simulink model "Sample594"  (R2021b)
settings: Solver=VariableStepAuto  StartTime=0.0  StopTime=10.0  RelTol=1e-3
undefined symbols (not defined in the file): DiscIntNeverNeededParam, magnitude, Newton, Raphson
libraries: simulink x402, pid_lib x98
(part 3 of 14)

== system Sample594/cfblk5/cfblk8/cfblk8 ==
  cfblk1 : Inport
  cfblk12 : Inport  Port=2
  cfblk10 : Subsystem
  cfblk11 : If  IfExpression=u1 >= 0  SampleTime=1
  cfblk13 : Subsystem  TreatAsAtomicUnit=on
  cfblk14 : Subsystem  TreatAsAtomicUnit=on
  cfblk{15..21} (7 alike) : Delay  SampleTime=1
  cfblk3 : simulink/Discrete/Difference  ICPrevInput=0.0  OutMin=[]  OutMax=[]  OutDataTypeStr=Inherit: Inherit via back propagation  OutDataType=fixdt(1, 16)  OutScaling=2^-10  DoSatur=off
  cfblk4 : UnitDelay  HasFrameUpgradeWarning=on
  cfblk5 : simulink/Discrete/Difference  ICPrevInput=0.0  OutMin=[]  OutMax=[]  OutDataTypeStr=Inherit: Inherit via back propagation  OutDataType=fixdt(1, 16)  OutScaling=2^-10  DoSatur=off
  cfblk6 : Gain  Gain=[-723830053.668321]
  cfblk7 : Reshape
  cfblk8 : Subsystem
  cfblk9 : Subsystem
  cfblk2 : Outport
  wires:
  cfblk13/1(cfblk2) -> cfblk6/1
  cfblk1/1 -> cfblk10/1(cfblk1)
  cfblk7/1 -> cfblk8/1(cfblk1)
  cfblk13/2(cfblk10) -> cfblk5/1
  cfblk8/1(cfblk2) -> cfblk4/1
  cfblk6/1 -> cfblk15/1, cfblk16/1, cfblk17/1
  cfblk13/3(cfblk11) -> cfblk2/1, cfblk7/1
  cfblk14/2(cfblk9) -> cfblk3/1
  cfblk10/1(cfblk2) -> cfblk9/2(cfblk12)
  cfblk12/1 -> cfblk14/2(cfblk8)
  cfblk3/1 -> cfblk8/2(cfblk7), cfblk21/1
  cfblk9/1(cfblk2) -> cfblk11/1, cfblk13/2(cfblk7)
  cfblk11/1 -> cfblk13/Action
  cfblk11/2 -> cfblk14/Action
  cfblk15/1 -> cfblk13/1(cfblk1)
  cfblk16/1 -> cfblk13/4(cfblk9)
  cfblk17/1 -> cfblk9/4(cfblk14)
  cfblk5/1 -> cfblk18/1
  cfblk18/1 -> cfblk14/1(cfblk1)
  cfblk14/1(cfblk2) -> cfblk19/1
  cfblk19/1 -> cfblk9/1(cfblk1)
  cfblk4/1 -> cfblk20/1
  cfblk20/1 -> cfblk9/3(cfblk13)
  cfblk21/1 -> cfblk13/3(cfblk8)

== system Sample594/cfblk6/cfblk10/cfblk6 ==
  cfblk1 : Inport
  cfblk12 : Inport  Port=2
  cfblk13 : Inport  Port=3
  cfblk14 : Inport  Port=4
  cfblk15 : Inport  Port=5
  cfblk10 : Subsystem
  cfblk11 : Subsystem
  cfblk{16..22} (7 alike) : Delay  SampleTime=1
  cfblk3 : PermuteDimensions
  cfblk4 : Subsystem
  cfblk5 : Subsystem
  cfblk6 : Subsystem
  cfblk7 : Subsystem
  cfblk8 : Subsystem
  cfblk9 : Subsystem
  cfblk2 : Outport
  wires:
  cfblk9/1(cfblk2) -> cfblk5/1(cfblk1)
  cfblk15/1 -> cfblk8/1(cfblk1)
  cfblk4/1(cfblk2) -> cfblk2/1
  cfblk8/1(cfblk2) -> cfblk6/1(cfblk1)
  cfblk12/1 -> cfblk4/1(cfblk1)
  cfblk1/1 -> cfblk9/2(cfblk13)
  cfblk13/1 -> cfblk7/1(cfblk1)
  cfblk3/1 -> cfblk4/2(cfblk11)
  cfblk8/2(cfblk11) -> cfblk10/1(cfblk1), cfblk6/6(cfblk17)
  cfblk14/1 -> cfblk4/3(cfblk12)
  cfblk5/2(cfblk14) -> cfblk7/2(cfblk11)
  cfblk6/1(cfblk2) -> cfblk10/3(cfblk6), cfblk11/3(cfblk14)
  cfblk10/1(cfblk2) -> cfblk3/1
  cfblk9/2(cfblk16) -> cfblk11/1(cfblk1)
  cfblk7/2(cfblk13) -> cfblk6/3(cfblk14)
  cfblk7/3(cfblk14) -> cfblk11/2(cfblk13)
  cfblk9/3(cfblk17) -> cfblk6/5(cfblk16), cfblk11/4(cfblk15)
  cfblk5/1(cfblk2) -> cfblk16/1
  cfblk16/1 -> cfblk9/3(cfblk14)
  cfblk7/1(cfblk2) -> cfblk17/1
  cfblk17/1 -> cfblk9/1(cfblk1)
  cfblk4/2(cfblk13) -> cfblk18/1
  cfblk18/1 -> cfblk10/2(cfblk5)
  cfblk10/2(cfblk7) -> cfblk19/1
  cfblk19/1 -> cfblk6/4(cfblk15)
  cfblk11/1(cfblk2) -> cfblk20/1
  cfblk20/1 -> cfblk6/2(cfblk13)
  cfblk11/2(cfblk16) -> cfblk21/1
  cfblk21/1 -> cfblk7/3(cfblk12)
  cfblk7/4(cfblk15) -> cfblk22/1
  cfblk22/1 -> cfblk9/4(cfblk15)

== system Sample594/cfblk6/cfblk10/cfblk7 ==
  cfblk1 : Inport
  cfblk10 : Inport  Port=2
  cfblk11 : Inport  Port=3
  cfblk13 : Delay  SampleTime=1
  cfblk3 : simulink/Discrete/Transfer Fcn Real Zero  ZeroZ=0.75  ICPrevInput=0.0  DoSatur=off
      settings: SourceProductBaseCode=SL
  cfblk4 : pid_lib/PID Controller  Controller=PID  Form=Parallel  TimeDomain=Discrete-time  UseExternalTs=off  SampleTime=1  IntegratorMethod=Forward Euler  FilterMethod=Forward Euler  ControllerParametersSource=internal  P=1  I=1  D=0  UseFilter=on  N=100  TunerSelectOption=Transfer Function Based (PID Tuner App)  InitialConditionSource=internal  InitialConditionForIntegrator=0  InitialConditionForFilter=0  DifferentiatorICPrevScaledInput=0  ExternalReset=none  TrackingMode=off  Kt=1  LimitOutput=off  SatLimitsSource=internal  UpperSaturationLimit=inf  LowerSaturationLimit=-inf  LinearizeAsGain=off  AntiWindupMode=none  Kb=1  POutMin=[]  POutMax=[]  IOutMin=[]  IOutMax=[]  DOutMin=[]  DOutMax=[]  NOutMin=[]  NOutMax=[]  SumOutMin=[]  SumOutMax=[]  SaturationOutMin=[]  SaturationOutMax=[]  PParamMin=[]  PParamMax=[]  IParamMin=[]  IParamMax=[]  DParamMin=[]  DParamMax=[]  NParamMin=[]  NParamMax=[]  KbParamMin=[]  KbParamMax=[]  KtParamMin=[]  KtParamMax=[]  KbOutMin=[]  KbOutMax=[]  KtOutMin=[]  KtOutMax=[]  IntegratorOutMin=[]  IntegratorOutMax=[]  FilterOutMin=[]  FilterOutMax=[]  SumI1OutMin=[]  SumI1OutMax=[]  SumI2OutMin=[]  SumI2OutMax=[]  SumI3OutMin=[]  SumI3OutMax=[]  SumI4OutMin=[]  SumI4OutMax=[]  SumDOutMin=[]  SumDOutMax=[]  DifferentiatorOutMin=[]  DifferentiatorOutMax=[]  FilterDiffOutCoefMin=[]  FilterDiffOutCoefMax=[]  ReciprocalOutMin=[]  ReciprocalOutMax=[]  SumDenOutMin=[]  SumDenOutMax=[]  SumNumOutMin=[]  SumNumOutMax=[]  DivideOutMin=[]  DivideOutMax=[]  UdiffTsProdOutMin=[]  UdiffTsProdOutMax=[]  NTsProdOutMin=[]  NTsProdOutMax=[]  UintegralTsProdOutMin=[]  UintegralTsProdOutMax=[]  UngainTsProdOutMin=[]  UngainTsProdOutMax=[]  IntegratorContinuousStateAttributes=''  IntegratorStateMustResolveToSignalObject=off  IntegratorRTWStateStorageClass=Auto  FilterContinuousStateAttributes=''  FilterStateMustResolveToSignalObject=off  FilterRTWStateStorageClass=Auto  ParallelPVariant=InternalParameters  IdealPVariant=Disabled  IVariant=InternalParameters  DVariant=InternalParameters  IntegratorVariant=Discrete  SatVariant=Disabled  AWVariant=Passthrough  PCopyVariant=Disabled  TRVariant=Disabled  FdbkBlocksVariant=Forward  IdealPFdbkVariant=Disabled  SatFdbkVariant=Disabled  DerivativeFilterVariant=ForwardEulerFilter  NVariant=InternalParameters  NCopyVariant=Disabled  FilterICVariant=InternalICsFilter  IntegratorICVariant=InternalICs  ExternalResetVariant=Disabled  TRSumVariant=Passthrough  SumFdbkVariant=Disabled  SumVariant=Sum_PID  TsampFilterVariant=InternalTs  TsampNgainVariant=Passthrough  TsampIntegralVariant=Passthrough  ExternalSaturationOutDataTypeStr=Inherit: Same as second input
  cfblk5 : ComplexToRealImag
  cfblk6 : Sqrt  SaturateOnIntegerOverflow=on
  cfblk7 : Subsystem
  cfblk8 : Subsystem
  cfblk9 : Subsystem
  cfblk2 : Outport
  cfblk12 : Outport  Port=2
  wires:
  cfblk3/1 -> cfblk6/1
  cfblk8/1(cfblk2) -> cfblk12/1
  cfblk5/1 -> cfblk4/1
  cfblk7/1(cfblk2) -> cfblk3/1
  cfblk1/1 -> cfblk5/1
  cfblk6/1 -> cfblk2/1
  cfblk10/1 -> cfblk7/1(cfblk1)
  cfblk9/1(cfblk2) -> cfblk7/2(cfblk6)
  cfblk11/1 -> cfblk8/1(cfblk1)
  cfblk4/1 -> cfblk9/1(cfblk1)
  cfblk5/2 -> cfblk9/2(cfblk10)
  cfblk7/2(cfblk7) -> cfblk13/1
  cfblk13/1 -> cfblk9/3(cfblk11)

== system Sample594/cfblk6/cfblk10/cfblk8 ==
  cfblk1 : Inport
  cfblk11 : Inport  Port=2
  cfblk10 : Subsystem
  cfblk12 : Delay  SampleTime=1
  cfblk13 : Delay  SampleTime=1
  cfblk3 : simulink/Discrete/Transfer Fcn First Order  PoleZ=0.95  ICPrevOutput=0.0  DoSatur=off
  cfblk4 : DotProduct  InputSameDT=on  OutDataTypeStr=Inherit: Inherit via internal rule
  cfblk5 : DotProduct  InputSameDT=on  OutDataTypeStr=Inherit: Inherit via internal rule
  cfblk6 : Sin  TimeSource=Use external signal  SampleTime=0
  cfblk7 : Constant  Value=[-545838641.656901]  SampleTime=1
  cfblk8 : Subsystem
  cfblk9 : Subsystem
  cfblk2 : Outport
  wires:
  cfblk1/1 -> cfblk3/1, cfblk5/2
  cfblk4/1 -> cfblk2/1
  cfblk11/1 -> cfblk4/1
  cfblk9/1(cfblk2) -> cfblk6/1
  cfblk5/1 -> cfblk4/2
  cfblk3/1 -> cfblk10/1(cfblk1)
  cfblk9/2(cfblk15) -> cfblk5/1
  cfblk10/1(cfblk2) -> cfblk8/1(cfblk1)
  cfblk8/1(cfblk2) -> cfblk9/1(cfblk1)
  cfblk7/1 -> cfblk10/3(cfblk14)
  cfblk10/2(cfblk15) -> cfblk9/2(cfblk14)
  cfblk6/1 -> cfblk12/1
  cfblk12/1 -> cfblk10/2(cfblk13)
  cfblk9/3(cfblk16) -> cfblk13/1
  cfblk13/1 -> cfblk8/2(cfblk9)

== system Sample594/cfblk6/cfblk11/cfblk10 ==
  cfblk1 : Inport
  cfblk8 : Inport  Port=2
  cfblk10 : Delay  SampleTime=1
  cfblk3 : DiscreteIntegrator  ICPrevOutput=DiscIntNeverNeededParam  ICPrevScaledInput=DiscIntNeverNeededParam
  cfblk4 : Signum
  cfblk5 : Subsystem
  cfblk6 : Subsystem
  cfblk7 : Subsystem
  cfblk9 : Delay  SampleTime=1
  cfblk2 : Outport
  wires:
  cfblk4/1 -> cfblk6/1(cfblk1)
  cfblk1/1 -> cfblk7/1(cfblk1), cfblk6/5(cfblk10)
  cfblk8/1 -> cfblk7/2(cfblk13)
  cfblk5/1(cfblk2) -> cfblk9/1, cfblk10/1
  cfblk7/1(cfblk2) -> cfblk4/1
  cfblk3/1 -> cfblk2/1
  cfblk7/2(cfblk15) -> cfblk6/2(cfblk7)
  cfblk6/1(cfblk2) -> cfblk3/1
  cfblk7/3(cfblk16) -> cfblk6/3(cfblk8)
  cfblk6/2(cfblk11) -> cfblk5/1(cfblk1)
  cfblk9/1 -> cfblk7/3(cfblk14)
  cfblk10/1 -> cfblk6/4(cfblk9)

== system Sample594/cfblk6/cfblk11/cfblk9 ==
  cfblk1 : Inport
  cfblk7 : Inport  Port=2
  cfblk3 : pid_lib/PID Controller  Controller=PID  Form=Parallel  TimeDomain=Discrete-time  UseExternalTs=off  SampleTime=1  IntegratorMethod=Forward Euler  FilterMethod=Forward Euler  ControllerParametersSource=internal  P=1  I=1  D=0  UseFilter=on  N=100  TunerSelectOption=Transfer Function Based (PID Tuner App)  InitialConditionSource=internal  InitialConditionForIntegrator=0  InitialConditionForFilter=0  DifferentiatorICPrevScaledInput=0  ExternalReset=none  TrackingMode=off  Kt=1  LimitOutput=off  SatLimitsSource=internal  UpperSaturationLimit=inf  LowerSaturationLimit=-inf  LinearizeAsGain=off  AntiWindupMode=none  Kb=1  POutMin=[]  POutMax=[]  IOutMin=[]  IOutMax=[]  DOutMin=[]  DOutMax=[]  NOutMin=[]  NOutMax=[]  SumOutMin=[]  SumOutMax=[]  SaturationOutMin=[]  SaturationOutMax=[]  PParamMin=[]  PParamMax=[]  IParamMin=[]  IParamMax=[]  DParamMin=[]  DParamMax=[]  NParamMin=[]  NParamMax=[]  KbParamMin=[]  KbParamMax=[]  KtParamMin=[]  KtParamMax=[]  KbOutMin=[]  KbOutMax=[]  KtOutMin=[]  KtOutMax=[]  IntegratorOutMin=[]  IntegratorOutMax=[]  FilterOutMin=[]  FilterOutMax=[]  SumI1OutMin=[]  SumI1OutMax=[]  SumI2OutMin=[]  SumI2OutMax=[]  SumI3OutMin=[]  SumI3OutMax=[]  SumI4OutMin=[]  SumI4OutMax=[]  SumDOutMin=[]  SumDOutMax=[]  DifferentiatorOutMin=[]  DifferentiatorOutMax=[]  FilterDiffOutCoefMin=[]  FilterDiffOutCoefMax=[]  ReciprocalOutMin=[]  ReciprocalOutMax=[]  SumDenOutMin=[]  SumDenOutMax=[]  SumNumOutMin=[]  SumNumOutMax=[]  DivideOutMin=[]  DivideOutMax=[]  UdiffTsProdOutMin=[]  UdiffTsProdOutMax=[]  NTsProdOutMin=[]  NTsProdOutMax=[]  UintegralTsProdOutMin=[]  UintegralTsProdOutMax=[]  UngainTsProdOutMin=[]  UngainTsProdOutMax=[]  IntegratorContinuousStateAttributes=''  IntegratorStateMustResolveToSignalObject=off  IntegratorRTWStateStorageClass=Auto  FilterContinuousStateAttributes=''  FilterStateMustResolveToSignalObject=off  FilterRTWStateStorageClass=Auto  ParallelPVariant=InternalParameters  IdealPVariant=Disabled  IVariant=InternalParameters  DVariant=InternalParameters  IntegratorVariant=Discrete  SatVariant=Disabled  AWVariant=Passthrough  PCopyVariant=Disabled  TRVariant=Disabled  FdbkBlocksVariant=Forward  IdealPFdbkVariant=Disabled  SatFdbkVariant=Disabled  DerivativeFilterVariant=ForwardEulerFilter  NVariant=InternalParameters  NCopyVariant=Disabled  FilterICVariant=InternalICsFilter  IntegratorICVariant=InternalICs  ExternalResetVariant=Disabled  TRSumVariant=Passthrough  SumFdbkVariant=Disabled  SumVariant=Sum_PID  TsampFilterVariant=InternalTs  TsampNgainVariant=Passthrough  TsampIntegralVariant=Passthrough  ExternalSaturationOutDataTypeStr=Inherit: Same as second input
  cfblk4 : Trigonometry
  cfblk5 : Constant  Value=[-699974006.887630]  SampleTime=1
  cfblk6 : Subsystem
  cfblk8 : Delay  SampleTime=1
  cfblk2 : Outport
  wires:
  cfblk7/1 -> cfblk2/1, cfblk6/3(cfblk7)
  cfblk5/1 -> cfblk6/1(cfblk1)
  cfblk3/1 -> cfblk4/1
  cfblk1/1 -> cfblk6/2(cfblk6)
  cfblk4/1 -> cfblk8/1
  cfblk8/1 -> cfblk3/1

== system Sample594/cfblk6/cfblk12/cfblk10 ==
  cfblk1 : Inport
  cfblk11 : Inport  Port=2
  cfblk10 : Rounding
  cfblk12 : Delay  SampleTime=1
  cfblk3 : simulink/Discrete/Transfer Fcn Lead or Lag  PoleZ=0.95  ZeroZ=0.75  ICPrevOutput=0.0  ICPrevInput=0.0  DoSatur=off
      settings: SourceProductBaseCode=SL
  cfblk4 : pid_lib/PID Controller (2DOF)  Controller=PID  Form=Parallel  TimeDomain=Discrete-time  UseExternalTs=off  SampleTime=1  IntegratorMethod=Forward Euler  FilterMethod=Forward Euler  ControllerParametersSource=internal  P=1  I=1  D=0  UseFilter=on  N=100  b=1  c=1  TunerSelectOption=Transfer Function Based (PID Tuner App)  InitialConditionSource=internal  InitialConditionForIntegrator=0  InitialConditionForFilter=0  DifferentiatorICPrevScaledInput=0  ExternalReset=none  TrackingMode=off  Kt=1  LimitOutput=off  SatLimitsSource=internal  UpperSaturationLimit=inf  LowerSaturationLimit=-inf  LinearizeAsGain=off  AntiWindupMode=none  Kb=1  POutMin=[]  POutMax=[]  IOutMin=[]  IOutMax=[]  DOutMin=[]  DOutMax=[]  NOutMin=[]  NOutMax=[]  bOutMin=[]  bOutMax=[]  cOutMin=[]  cOutMax=[]  SumOutMin=[]  SumOutMax=[]  SaturationOutMin=[]  SaturationOutMax=[]  PParamMin=[]  PParamMax=[]  IParamMin=[]  IParamMax=[]  DParamMin=[]  DParamMax=[]  NParamMin=[]  NParamMax=[]  bParamMin=[]  bParamMax=[]  cParamMin=[]  cParamMax=[]  KbParamMin=[]  KbParamMax=[]  KtParamMin=[]  KtParamMax=[]  KbOutMin=[]  KbOutMax=[]  KtOutMin=[]  KtOutMax=[]  IntegratorOutMin=[]  IntegratorOutMax=[]  FilterOutMin=[]  FilterOutMax=[]  SumI1OutMin=[]  SumI1OutMax=[]  SumI2OutMin=[]  SumI2OutMax=[]  SumI3OutMin=[]  SumI3OutMax=[]  SumI4OutMin=[]  SumI4OutMax=[]  SumDOutMin=[]  SumDOutMax=[]  Sum1OutMin=[]  Sum1OutMax=[]  Sum2OutMin=[]  Sum2OutMax=[]  Sum3OutMin=[]  Sum3OutMax=[]  DifferentiatorOutMin=[]  DifferentiatorOutMax=[]  FilterDiffOutCoefMin=[]  FilterDiffOutCoefMax=[]  ReciprocalOutMin=[]  ReciprocalOutMax=[]  SumDenOutMin=[]  SumDenOutMax=[]  SumNumOutMin=[]  SumNumOutMax=[]  DivideOutMin=[]  DivideOutMax=[]  UdiffTsProdOutMin=[]  UdiffTsProdOutMax=[]  NTsProdOutMin=[]  NTsProdOutMax=[]  UintegralTsProdOutMin=[]  UintegralTsProdOutMax=[]  UngainTsProdOutMin=[]  UngainTsProdOutMax=[]  IntegratorContinuousStateAttributes=''  IntegratorStateMustResolveToSignalObject=off  IntegratorRTWStateStorageClass=Auto  FilterContinuousStateAttributes=''  FilterStateMustResolveToSignalObject=off  FilterRTWStateStorageClass=Auto  ParallelPVariant=InternalParameters  IdealPVariant=Disabled  IVariant=InternalParameters  DVariant=InternalParameters  bVariant=InternalParameters  cVariant=InternalParameters  IntegratorVariant=Discrete  SatVariant=Disabled  AWVariant=Passthrough  PCopyVariant=Disabled  TRVariant=Disabled  FdbkBlocksVariant=Forward  IdealPFdbkVariant=Disabled  SatFdbkVariant=Disabled  DerivativeFilterVariant=ForwardEulerFilter  NVariant=InternalParameters  NCopyVariant=Disabled  FilterICVariant=InternalICsFilter  IntegratorICVariant=InternalICs  ExternalResetVariant=Disabled  TRSumVariant=Passthrough  SumFdbkVariant=Disabled  SumVariant=Sum_PID  TsampFilterVariant=InternalTs  TsampNgainVariant=Passthrough  TsampIntegralVariant=Passthrough  ExternalSaturationOutDataTypeStr=Inherit: Same as second input
      settings: SourceProductBaseCode=SL
  cfblk5 : Sum  Inputs=|++
  cfblk6 : Product  Inputs=**
  cfblk7 : Reshape
  cfblk8 : ComplexToMagnitudeAngle
  cfblk9 : Reshape
  cfblk2 : Outport
  wires:
  cfblk5/1 -> cfblk3/1
  cfblk9/1 -> cfblk7/1, cfblk5/2
  cfblk1/1 -> cfblk10/1
  cfblk6/1 -> cfblk8/1
  cfblk11/1 -> cfblk9/1
  cfblk7/1 -> cfblk4/1
  cfblk4/1 -> cfblk2/1
  cfblk3/1 -> cfblk6/1
  cfblk10/1 -> cfblk5/1
  cfblk8/2 -> cfblk4/2
  cfblk8/1 -> cfblk12/1
  cfblk12/1 -> cfblk6/2

== system Sample594/cfblk6/cfblk12/cfblk9 ==
  cfblk1 : Inport
  cfblk{10..14} (5 alike) : Delay  SampleTime=1
  cfblk3 : Delay  DelayLengthSource=Input port  SampleTime=1
      settings: InputPortMap=u0,p1
  cfblk4 : pid_lib/PID Controller  Controller=PID  Form=Parallel  TimeDomain=Discrete-time  UseExternalTs=off  SampleTime=1  IntegratorMethod=Forward Euler  FilterMethod=Forward Euler  ControllerParametersSource=internal  P=1  I=1  D=0  UseFilter=on  N=100  TunerSelectOption=Transfer Function Based (PID Tuner App)  InitialConditionSource=internal  InitialConditionForIntegrator=0  InitialConditionForFilter=0  DifferentiatorICPrevScaledInput=0  ExternalReset=none  TrackingMode=off  Kt=1  LimitOutput=off  SatLimitsSource=internal  UpperSaturationLimit=inf  LowerSaturationLimit=-inf  LinearizeAsGain=off  AntiWindupMode=none  Kb=1  POutMin=[]  POutMax=[]  IOutMin=[]  IOutMax=[]  DOutMin=[]  DOutMax=[]  NOutMin=[]  NOutMax=[]  SumOutMin=[]  SumOutMax=[]  SaturationOutMin=[]  SaturationOutMax=[]  PParamMin=[]  PParamMax=[]  IParamMin=[]  IParamMax=[]  DParamMin=[]  DParamMax=[]  NParamMin=[]  NParamMax=[]  KbParamMin=[]  KbParamMax=[]  KtParamMin=[]  KtParamMax=[]  KbOutMin=[]  KbOutMax=[]  KtOutMin=[]  KtOutMax=[]  IntegratorOutMin=[]  IntegratorOutMax=[]  FilterOutMin=[]  FilterOutMax=[]  SumI1OutMin=[]  SumI1OutMax=[]  SumI2OutMin=[]  SumI2OutMax=[]  SumI3OutMin=[]  SumI3OutMax=[]  SumI4OutMin=[]  SumI4OutMax=[]  SumDOutMin=[]  SumDOutMax=[]  DifferentiatorOutMin=[]  DifferentiatorOutMax=[]  FilterDiffOutCoefMin=[]  FilterDiffOutCoefMax=[]  ReciprocalOutMin=[]  ReciprocalOutMax=[]  SumDenOutMin=[]  SumDenOutMax=[]  SumNumOutMin=[]  SumNumOutMax=[]  DivideOutMin=[]  DivideOutMax=[]  UdiffTsProdOutMin=[]  UdiffTsProdOutMax=[]  NTsProdOutMin=[]  NTsProdOutMax=[]  UintegralTsProdOutMin=[]  UintegralTsProdOutMax=[]  UngainTsProdOutMin=[]  UngainTsProdOutMax=[]  IntegratorContinuousStateAttributes=''  IntegratorStateMustResolveToSignalObject=off  IntegratorRTWStateStorageClass=Auto  FilterContinuousStateAttributes=''  FilterStateMustResolveToSignalObject=off  FilterRTWStateStorageClass=Auto  ParallelPVariant=InternalParameters  IdealPVariant=Disabled  IVariant=InternalParameters  DVariant=InternalParameters  IntegratorVariant=Discrete  SatVariant=Disabled  AWVariant=Passthrough  PCopyVariant=Disabled  TRVariant=Disabled  FdbkBlocksVariant=Forward  IdealPFdbkVariant=Disabled  SatFdbkVariant=Disabled  DerivativeFilterVariant=ForwardEulerFilter  NVariant=InternalParameters  NCopyVariant=Disabled  FilterICVariant=InternalICsFilter  IntegratorICVariant=InternalICs  ExternalResetVariant=Disabled  TRSumVariant=Passthrough  SumFdbkVariant=Disabled  SumVariant=Sum_PID  TsampFilterVariant=InternalTs  TsampNgainVariant=Passthrough  TsampIntegralVariant=Passthrough  ExternalSaturationOutDataTypeStr=Inherit: Same as second input
  cfblk5 : MinMax  Function=max  Inputs=3
  cfblk6 : Subsystem
  cfblk7 : Subsystem
  cfblk8 : Subsystem
  cfblk9 : Subsystem
  cfblk2 : Outport
  wires:
  cfblk5/1 -> cfblk7/1(cfblk1), cfblk7/3(cfblk11)
  cfblk1/1 -> cfblk9/2(cfblk12), cfblk6/2(cfblk13)
  cfblk6/1(cfblk2) -> cfblk8/1(cfblk1)
  cfblk3/1 -> cfblk6/1(cfblk1)
  cfblk9/1(cfblk2) -> cfblk5/1, cfblk5/2
  cfblk4/1 -> cfblk3/1, cfblk14/1
  cfblk7/2(cfblk12) -> cfblk4/1, cfblk8/4(cfblk11), cfblk6/3(cfblk14)
  cfblk6/2(cfblk15) -> cfblk8/2(cfblk9)
  cfblk6/3(cfblk16) -> cfblk2/1
  cfblk6/4(cfblk17) -> cfblk8/3(cfblk10), cfblk8/5(cfblk12), cfblk13/1
  cfblk7/1(cfblk2) -> cfblk10/1
  cfblk10/1 -> cfblk9/1(cfblk1)
  cfblk8/1(cfblk2) -> cfblk11/1
  cfblk11/1 -> cfblk3/2
  cfblk8/2(cfblk13) -> cfblk12/1
  cfblk12/1 -> cfblk9/3(cfblk13)
  cfblk13/1 -> cfblk5/3
  cfblk14/1 -> cfblk7/2(cfblk10)

== system Sample594/cfblk6/cfblk7/cfblk5 ==
  cfblk1 : Inport
  cfblk10 : Subsystem
  cfblk{3,12..14} (4 alike) : Delay  SampleTime=1
  cfblk4 : pid_lib/PID Controller (2DOF)  Controller=PID  Form=Parallel  TimeDomain=Discrete-time  UseExternalTs=off  SampleTime=1  IntegratorMethod=Forward Euler  FilterMethod=Forward Euler  ControllerParametersSource=internal  P=1  I=1  D=0  UseFilter=on  N=100  b=1  c=1  TunerSelectOption=Transfer Function Based (PID Tuner App)  InitialConditionSource=internal  InitialConditionForIntegrator=0  InitialConditionForFilter=0  DifferentiatorICPrevScaledInput=0  ExternalReset=none  TrackingMode=off  Kt=1  LimitOutput=off  SatLimitsSource=internal  UpperSaturationLimit=inf  LowerSaturationLimit=-inf  LinearizeAsGain=off  AntiWindupMode=none  Kb=1  POutMin=[]  POutMax=[]  IOutMin=[]  IOutMax=[]  DOutMin=[]  DOutMax=[]  NOutMin=[]  NOutMax=[]  bOutMin=[]  bOutMax=[]  cOutMin=[]  cOutMax=[]  SumOutMin=[]  SumOutMax=[]  SaturationOutMin=[]  SaturationOutMax=[]  PParamMin=[]  PParamMax=[]  IParamMin=[]  IParamMax=[]  DParamMin=[]  DParamMax=[]  NParamMin=[]  NParamMax=[]  bParamMin=[]  bParamMax=[]  cParamMin=[]  cParamMax=[]  KbParamMin=[]  KbParamMax=[]  KtParamMin=[]  KtParamMax=[]  KbOutMin=[]  KbOutMax=[]  KtOutMin=[]  KtOutMax=[]  IntegratorOutMin=[]  IntegratorOutMax=[]  FilterOutMin=[]  FilterOutMax=[]  SumI1OutMin=[]  SumI1OutMax=[]  SumI2OutMin=[]  SumI2OutMax=[]  SumI3OutMin=[]  SumI3OutMax=[]  SumI4OutMin=[]  SumI4OutMax=[]  SumDOutMin=[]  SumDOutMax=[]  Sum1OutMin=[]  Sum1OutMax=[]  Sum2OutMin=[]  Sum2OutMax=[]  Sum3OutMin=[]  Sum3OutMax=[]  DifferentiatorOutMin=[]  DifferentiatorOutMax=[]  FilterDiffOutCoefMin=[]  FilterDiffOutCoefMax=[]  ReciprocalOutMin=[]  ReciprocalOutMax=[]  SumDenOutMin=[]  SumDenOutMax=[]  SumNumOutMin=[]  SumNumOutMax=[]  DivideOutMin=[]  DivideOutMax=[]  UdiffTsProdOutMin=[]  UdiffTsProdOutMax=[]  NTsProdOutMin=[]  NTsProdOutMax=[]  UintegralTsProdOutMin=[]  UintegralTsProdOutMax=[]  UngainTsProdOutMin=[]  UngainTsProdOutMax=[]  IntegratorContinuousStateAttributes=''  IntegratorStateMustResolveToSignalObject=off  IntegratorRTWStateStorageClass=Auto  FilterContinuousStateAttributes=''  FilterStateMustResolveToSignalObject=off  FilterRTWStateStorageClass=Auto  ParallelPVariant=InternalParameters  IdealPVariant=Disabled  IVariant=InternalParameters  DVariant=InternalParameters  bVariant=InternalParameters  cVariant=InternalParameters  IntegratorVariant=Discrete  SatVariant=Disabled  AWVariant=Passthrough  PCopyVariant=Disabled  TRVariant=Disabled  FdbkBlocksVariant=Forward  IdealPFdbkVariant=Disabled  SatFdbkVariant=Disabled  DerivativeFilterVariant=ForwardEulerFilter  NVariant=InternalParameters  NCopyVariant=Disabled  FilterICVariant=InternalICsFilter  IntegratorICVariant=InternalICs  ExternalResetVariant=Disabled  TRSumVariant=Passthrough  SumFdbkVariant=Disabled  SumVariant=Sum_PID  TsampFilterVariant=InternalTs  TsampNgainVariant=Passthrough  TsampIntegralVariant=Passthrough  ExternalSaturationOutDataTypeStr=Inherit: Same as second input
      settings: SourceProductBaseCode=SL
  cfblk5 : Signum
  cfblk6 : Constant  Value=[523165528.217470]  SampleTime=1
  cfblk7 : Subsystem
  cfblk8 : Subsystem
  cfblk9 : Subsystem
  cfblk2 : Outport
  cfblk11 : Outport  Port=2
  wires:
  cfblk8/1(cfblk2) -> cfblk10/1(cfblk1), cfblk7/3(cfblk13), cfblk9/2(cfblk13), cfblk4/2
  cfblk3/1 -> cfblk9/1(cfblk1)
  cfblk6/1 -> cfblk11/1
  cfblk10/1(cfblk2) -> cfblk3/1, cfblk7/5(cfblk15)
  cfblk1/1 -> cfblk2/1, cfblk8/3(cfblk7)
  cfblk9/1(cfblk2) -> cfblk5/1
  cfblk9/2(cfblk14) -> cfblk7/1(cfblk1), cfblk7/4(cfblk14)
  cfblk5/1 -> cfblk7/2(cfblk12)
  cfblk7/1(cfblk2) -> cfblk4/1
  cfblk4/1 -> cfblk12/1
  cfblk12/1 -> cfblk8/2(cfblk6)
  cfblk7/2(cfblk16) -> cfblk13/1
  cfblk13/1 -> cfblk10/2(cfblk11)
  cfblk7/3(cfblk17) -> cfblk14/1
  cfblk14/1 -> cfblk8/1(cfblk1)

== system Sample594/cfblk6/cfblk7/cfblk6 ==
  cfblk1 : Inport
  cfblk12 : Inport  Port=2
  cfblk13 : Inport  Port=3
  cfblk10 : Subsystem
  cfblk11 : Subsystem
  cfblk{14..22} (9 alike) : Delay  SampleTime=1
  cfblk3 : simulink/Math Operations/Slider Gain  gain=1  low=0  high=2
  cfblk4 : MinMax  Inputs=2
  cfblk5 : Sum  Inputs=+-
  cfblk6 : Sum  Inputs=|++
  cfblk7 : Sum  Inputs=+-
  cfblk8 : Subsystem
  cfblk9 : Subsystem
  cfblk2 : Outport
  wires:
  cfblk10/1(cfblk2) -> cfblk5/1, cfblk9/2(cfblk9)
  cfblk8/1(cfblk2) -> cfblk6/1
  cfblk3/1 -> cfblk4/1, cfblk8/1(cfblk1), cfblk22/1
  cfblk8/2(cfblk8) -> cfblk4/2
  cfblk5/1 -> cfblk14/1, cfblk15/1
  cfblk9/1(cfblk2) -> cfblk3/1
  cfblk6/1 -> cfblk7/1
  cfblk7/1 -> cfblk17/1, cfblk18/1, cfblk19/1, cfblk20/1
  cfblk13/1 -> cfblk7/2, cfblk9/1(cfblk1), cfblk10/8(cfblk15)
  cfblk9/2(cfblk13) -> cfblk6/2
  cfblk4/1 -> cfblk5/2, cfblk16/1
  cfblk12/1 -> cfblk2/1
  cfblk1/1 -> cfblk11/2(cfblk8), cfblk10/7(cfblk14)
  cfblk11/1(cfblk2) -> cfblk10/3(cfblk10), cfblk9/4(cfblk11)
  cfblk14/1 -> cfblk10/1(cfblk1)
  cfblk15/1 -> cfblk11/3(cfblk9)
  cfblk16/1 -> cfblk10/5(cfblk12)
  cfblk17/1 -> cfblk10/2(cfblk9)
  cfblk18/1 -> cfblk10/4(cfblk11)
  cfblk19/1 -> cfblk10/6(cfblk13)
  cfblk20/1 -> cfblk9/5(cfblk12)
  cfblk8/3(cfblk9) -> cfblk21/1
  cfblk21/1 -> cfblk11/1(cfblk1)
  cfblk22/1 -> cfblk9/3(cfblk10)

== system Sample594/cfblk6/cfblk8/cfblk10 ==
  cfblk1 : Inport
  cfblk3 : DiscreteFir  SampleTime=1
  cfblk4 : simulink/Discrete/Transfer Fcn Real Zero  ZeroZ=0.75  ICPrevInput=0.0  DoSatur=off
      settings: SourceProductBaseCode=SL
  cfblk5 : Sqrt  Operator=rSqrt  AlgorithmType=Newton-Raphson  SaturateOnIntegerOverflow=on
  cfblk6 : DotProduct  InputSameDT=on  OutDataTypeStr=Inherit: Inherit via internal rule
  cfblk7 : Constant  Value=[-681644518.584127]  SampleTime=1
  cfblk8 : Subsystem
  cfblk2 : Outport
  cfblk9 : Outport  Port=2
  wires:
  cfblk5/1 -> cfblk8/1(cfblk1)
  cfblk3/1 -> cfblk5/1
  cfblk6/1 -> cfblk3/1
  cfblk4/1 -> cfblk9/1
  cfblk7/1 -> cfblk6/1
  cfblk8/1(cfblk2) -> cfblk4/1
  cfblk8/2(cfblk13) -> cfblk2/1
  cfblk1/1 -> cfblk6/2

== system Sample594/cfblk6/cfblk8/cfblk11 ==
  cfblk1 : Inport
  cfblk8 : Inport  Port=2
  cfblk9 : Inport  Port=3
  cfblk3 : ComplexToMagnitudeAngle
  cfblk4 : Math  Operator=log10  SaturateOnIntegerOverflow=on
  cfblk5 : Constant  Value=[843527687.838584]  SampleTime=1
  cfblk6 : Constant  Value=[882982120.415271]  SampleTime=1
  cfblk7 : Subsystem
  cfblk2 : Outport
  wires:
  cfblk1/1 -> cfblk7/1(cfblk1)
  cfblk9/1 -> cfblk4/1
  cfblk7/1(cfblk2) -> cfblk3/1
  cfblk3/1 -> cfblk2/1

== system Sample594/cfblk6/cfblk9/cfblk10 ==
  cfblk1 : Inport
  cfblk13 : Inport  Port=2
  cfblk14 : Inport  Port=3
  cfblk10 : ComplexToRealImag
  cfblk11 : Subsystem
  cfblk12 : Subsystem
  cfblk16 : Delay  SampleTime=1
  cfblk17 : Delay  SampleTime=1
  cfblk3 : DiscreteFilter  SampleTime=1
  cfblk4 : Product  Inputs=**
  cfblk5 : DotProduct  InputSameDT=on  OutDataTypeStr=Inherit: Inherit via internal rule
  cfblk6 : ComplexToMagnitudeAngle
  cfblk7 : Sqrt  Operator=rSqrt  AlgorithmType=Newton-Raphson  SaturateOnIntegerOverflow=on
  cfblk8 : Rounding
  cfblk9 : Math  Operator=mod  SaturateOnIntegerOverflow=on
  cfblk2 : Outport
  cfblk15 : Outport  Port=2
  wires:
  cfblk13/1 -> cfblk11/1(cfblk1)
  cfblk11/1(cfblk2) -> cfblk9/1
  cfblk4/1 -> cfblk3/1
  cfblk8/1 -> cfblk2/1
  cfblk11/3(cfblk9) -> cfblk6/1
  cfblk5/1 -> cfblk4/1
  cfblk10/1 -> cfblk11/2(cfblk7)
  cfblk1/1 -> cfblk5/1
  cfblk6/1 -> cfblk7/1
  cfblk14/1 -> cfblk9/2
  cfblk12/1(cfblk2) -> cfblk15/1
  cfblk7/1 -> cfblk5/2, cfblk12/3(cfblk10)
  cfblk9/1 -> cfblk12/1(cfblk1)
  cfblk6/2 -> cfblk8/1
  cfblk10/2 -> cfblk12/2(cfblk9)
  cfblk3/1 -> cfblk16/1
  cfblk16/1 -> cfblk4/2
  cfblk11/2(cfblk8) -> cfblk17/1
  cfblk17/1 -> cfblk10/1

== system Sample594/cfblk6/cfblk9/cfblk11 ==
  cfblk1 : Inport
  cfblk8 : Inport  Port=2
  cfblk9 : Inport  Port=3
  cfblk3 : DiscreteFir  SampleTime=1
  cfblk4 : Polyval  Coefs=[ +2.081618890e-019, -1.441693666e-014, +4.719686976e-010, -8.536869453e-006, +1.621573104e-001, -8.087801117e+001 ]
  cfblk5 : Sin  TimeSource=Use external signal  SampleTime=0
  cfblk6 : Math  Operator=conj  SaturateOnIntegerOverflow=on
  cfblk7 : Sqrt  Operator=rSqrt  AlgorithmType=Newton-Raphson  SaturateOnIntegerOverflow=on
  cfblk2 : Outport
  cfblk10 : Outport  Port=2
  wires:
  cfblk3/1 -> cfblk5/1
  cfblk4/1 -> cfblk3/1
  cfblk6/1 -> cfblk4/1
  cfblk8/1 -> cfblk6/1
  cfblk5/1 -> cfblk10/1
  cfblk9/1 -> cfblk7/1
  cfblk1/1 -> cfblk2/1

== system Sample594/cfblk6/cfblk9/cfblk12 ==
  cfblk1 : Inport
  cfblk7 : Inport  Port=2
  cfblk8 : Inport  Port=3
  cfblk3 : simulink/Discrete/Tapped Delay  vinit=0.0  samptime=-1  NumDelays=1  DelayOrder=Oldest  includeCurrent=off
  cfblk4 : DiscreteIntegrator  ICPrevOutput=DiscIntNeverNeededParam  ICPrevScaledInput=DiscIntNeverNeededParam
  cfblk5 : Subsystem
  cfblk6 : Subsystem
  cfblk2 : Outport
  cfblk9 : Outport  Port=2
  wires:
  cfblk1/1 -> cfblk4/1
  cfblk7/1 -> cfblk5/1(cfblk1)
  cfblk8/1 -> cfblk2/1, cfblk6/2(cfblk6)
  cfblk4/1 -> cfblk3/1, cfblk6/3(cfblk7)
  cfblk3/1 -> cfblk5/2(cfblk9), cfblk6/1(cfblk1)
  cfblk6/1(cfblk2) -> cfblk5/3(cfblk10)
  cfblk5/1(cfblk2) -> cfblk9/1
  cfblk6/2(cfblk8) -> cfblk5/4(cfblk11)

== system Sample594/cfblk6/cfblk9/cfblk13 ==
  cfblk1 : Inport
  cfblk10 : Delay  SampleTime=1
  cfblk11 : Delay  SampleTime=1
  cfblk12 : Delay  SampleTime=1
  cfblk3 : simulink/Discrete/Transfer Fcn First Order  PoleZ=0.95  ICPrevOutput=0.0  DoSatur=off
  cfblk4 : Product  Inputs=**
  cfblk5 : Sin  TimeSource=Use external signal  SampleTime=0
  cfblk6 : Rounding
  cfblk7 : Subsystem
  cfblk8 : Subsystem
  cfblk9 : Subsystem
  cfblk2 : Outport
  wires:
  cfblk8/1(cfblk2) -> cfblk4/1
  cfblk4/1 -> cfblk3/1
  cfblk1/1 -> cfblk5/1
  cfblk3/1 -> cfblk7/2(cfblk11), cfblk2/1
  cfblk8/2(cfblk13) -> cfblk9/1(cfblk1)
  cfblk7/2(cfblk12) -> cfblk9/2(cfblk11), cfblk6/1
  cfblk5/1 -> cfblk8/2(cfblk12)
  cfblk7/1(cfblk2) -> cfblk10/1
  cfblk10/1 -> cfblk4/2
  cfblk9/1(cfblk2) -> cfblk11/1
  cfblk11/1 -> cfblk7/1(cfblk1)
  cfblk6/1 -> cfblk12/1
  cfblk12/1 -> cfblk8/1(cfblk1)

== system Sample594/cfblk6/cfblk9/cfblk8 ==
  cfblk1 : Inport
  cfblk11 : Inport  Port=2
  cfblk12 : Inport  Port=3
  cfblk10 : Subsystem
  cfblk14 : Delay  SampleTime=1
  cfblk3 : Math  Operator=hypot  SaturateOnIntegerOverflow=on
  cfblk4 : Reshape
  cfblk5 : Sum  Inputs=|++
  cfblk6 : Reshape
  cfblk7 : Gain  Gain=[701799016.262811]
  cfblk8 : Subsystem
  cfblk9 : Subsystem
  cfblk2 : Outport
  cfblk13 : Outport  Port=2
  wires:
  cfblk10/1(cfblk2) -> cfblk9/1(cfblk1), cfblk8/4(cfblk11)
  cfblk9/1(cfblk2) -> cfblk6/1
  cfblk5/1 -> cfblk10/1(cfblk1)
  cfblk12/1 -> cfblk5/1, cfblk10/2(cfblk9)
  cfblk3/1 -> cfblk5/2
  cfblk8/1(cfblk2) -> cfblk7/1
  cfblk8/2(cfblk12) -> cfblk4/1
  cfblk11/1 -> cfblk9/2(cfblk10), cfblk8/3(cfblk10)
  cfblk1/1 -> cfblk3/1, cfblk9/3(cfblk11)
  cfblk7/1 -> cfblk2/1
  cfblk6/1 -> cfblk8/1(cfblk1)
  cfblk4/1 -> cfblk13/1, cfblk14/1
  cfblk9/2(cfblk12) -> cfblk8/2(cfblk9)
  cfblk14/1 -> cfblk3/2

== system Sample594/cfblk6/cfblk9/cfblk9 ==
  cfblk1 : Inport
  cfblk7 : Inport  Port=2
  cfblk8 : Inport  Port=3
  cfblk10 : Delay  SampleTime=1
  cfblk3 : Delay  ShowEnablePort=on  SampleTime=1
      settings: InputPortMap=u0,e6
  cfblk4 : Signum
  cfblk5 : Squeeze
  cfblk6 : Subsystem
  cfblk9 : Delay  SampleTime=1
  cfblk2 : Outport
  wires:
  cfblk1/1 -> cfblk3/1, cfblk6/5(cfblk16)
  cfblk7/1 -> cfblk6/2(cfblk13)
  cfblk8/1 -> cfblk6/3(cfblk14)
  cfblk3/1 -> cfblk6/4(cfblk15)
  cfblk6/1(cfblk2) -> cfblk2/1
  cfblk6/2(cfblk17) -> cfblk5/1, cfblk4/1
  cfblk5/1 -> cfblk9/1
  cfblk9/1 -> cfblk6/1(cfblk1)
  cfblk4/1 -> cfblk10/1
  cfblk10/1 -> cfblk3/2

== system Sample594/cfblk7/cfblk10/cfblk10 ==
  cfblk1 : Inport
  cfblk12 : Inport  Port=2
  cfblk13 : Inport  Port=3
  cfblk10 : Subsystem
  cfblk11 : Subsystem
  cfblk18 : Delay  SampleTime=1
  cfblk19 : Delay  SampleTime=1
  cfblk3 : DiscreteStateSpace
  cfblk4 : pid_lib/PID Controller (2DOF)  Controller=PID  Form=Parallel  TimeDomain=Discrete-time  UseExternalTs=off  SampleTime=1  IntegratorMethod=Forward Euler  FilterMethod=Forward Euler  ControllerParametersSource=internal  P=1  I=1  D=0  UseFilter=on  N=100  b=1  c=1  TunerSelectOption=Transfer Function Based (PID Tuner App)  InitialConditionSource=internal  InitialConditionForIntegrator=0  InitialConditionForFilter=0  DifferentiatorICPrevScaledInput=0  ExternalReset=none  TrackingMode=off  Kt=1  LimitOutput=off  SatLimitsSource=internal  UpperSaturationLimit=inf  LowerSaturationLimit=-inf  LinearizeAsGain=off  AntiWindupMode=none  Kb=1  POutMin=[]  POutMax=[]  IOutMin=[]  IOutMax=[]  DOutMin=[]  DOutMax=[]  NOutMin=[]  NOutMax=[]  bOutMin=[]  bOutMax=[]  cOutMin=[]  cOutMax=[]  SumOutMin=[]  SumOutMax=[]  SaturationOutMin=[]  SaturationOutMax=[]  PParamMin=[]  PParamMax=[]  IParamMin=[]  IParamMax=[]  DParamMin=[]  DParamMax=[]  NParamMin=[]  NParamMax=[]  bParamMin=[]  bParamMax=[]  cParamMin=[]  cParamMax=[]  KbParamMin=[]  KbParamMax=[]  KtParamMin=[]  KtParamMax=[]  KbOutMin=[]  KbOutMax=[]  KtOutMin=[]  KtOutMax=[]  IntegratorOutMin=[]  IntegratorOutMax=[]  FilterOutMin=[]  FilterOutMax=[]  SumI1OutMin=[]  SumI1OutMax=[]  SumI2OutMin=[]  SumI2OutMax=[]  SumI3OutMin=[]  SumI3OutMax=[]  SumI4OutMin=[]  SumI4OutMax=[]  SumDOutMin=[]  SumDOutMax=[]  Sum1OutMin=[]  Sum1OutMax=[]  Sum2OutMin=[]  Sum2OutMax=[]  Sum3OutMin=[]  Sum3OutMax=[]  DifferentiatorOutMin=[]  DifferentiatorOutMax=[]  FilterDiffOutCoefMin=[]  FilterDiffOutCoefMax=[]  ReciprocalOutMin=[]  ReciprocalOutMax=[]  SumDenOutMin=[]  SumDenOutMax=[]  SumNumOutMin=[]  SumNumOutMax=[]  DivideOutMin=[]  DivideOutMax=[]  UdiffTsProdOutMin=[]  UdiffTsProdOutMax=[]  NTsProdOutMin=[]  NTsProdOutMax=[]  UintegralTsProdOutMin=[]  UintegralTsProdOutMax=[]  UngainTsProdOutMin=[]  UngainTsProdOutMax=[]  IntegratorContinuousStateAttributes=''  IntegratorStateMustResolveToSignalObject=off  IntegratorRTWStateStorageClass=Auto  FilterContinuousStateAttributes=''  FilterStateMustResolveToSignalObject=off  FilterRTWStateStorageClass=Auto  ParallelPVariant=InternalParameters  IdealPVariant=Disabled  IVariant=InternalParameters  DVariant=InternalParameters  bVariant=InternalParameters  cVariant=InternalParameters  IntegratorVariant=Discrete  SatVariant=Disabled  AWVariant=Passthrough  PCopyVariant=Disabled  TRVariant=Disabled  FdbkBlocksVariant=Forward  IdealPFdbkVariant=Disabled  SatFdbkVariant=Disabled  DerivativeFilterVariant=ForwardEulerFilter  NVariant=InternalParameters  NCopyVariant=Disabled  FilterICVariant=InternalICsFilter  IntegratorICVariant=InternalICs  ExternalResetVariant=Disabled  TRSumVariant=Passthrough  SumFdbkVariant=Disabled  SumVariant=Sum_PID  TsampFilterVariant=InternalTs  TsampNgainVariant=Passthrough  TsampIntegralVariant=Passthrough  ExternalSaturationOutDataTypeStr=Inherit: Same as second input
      settings: SourceProductBaseCode=SL
  cfblk5 : PermuteDimensions
  cfblk6 : Trigonometry
  cfblk7 : Constant  Value=[-87159574.439061]  SampleTime=1
  cfblk8 : Subsystem
  cfblk9 : Subsystem
  cfblk2 : Outport
  cfblk14 : Outport  Port=2
  cfblk15 : Outport  Port=3
  cfblk16 : Outport  Port=4
  cfblk17 : Outport  Port=5
  wires:
  cfblk1/1 -> cfblk9/1(cfblk1)
  cfblk10/1(cfblk2) -> cfblk17/1
  cfblk6/1 -> cfblk2/1, cfblk10/2(cfblk10)
  cfblk9/1(cfblk2) -> cfblk14/1, cfblk4/2, cfblk15/1, cfblk10/3(cfblk11)
  cfblk7/1 -> cfblk9/2(cfblk5), cfblk10/1(cfblk1), cfblk11/3(cfblk13), cfblk11/4(cfblk14)
  cfblk3/1 -> cfblk5/1, cfblk11/2(cfblk12)
  cfblk8/1(cfblk2) -> cfblk11/5(cfblk15), cfblk19/1
  cfblk5/1 -> cfblk16/1
  cfblk10/2(cfblk12) -> cfblk8/1(cfblk1)
  cfblk12/1 -> cfblk4/1
  cfblk4/1 -> cfblk3/1, cfblk6/1
  cfblk13/1 -> cfblk11/1(cfblk1)
  cfblk11/1(cfblk2) -> cfblk18/1
  cfblk18/1 -> cfblk9/4(cfblk7)
  cfblk19/1 -> cfblk9/3(cfblk6)

== system Sample594/cfblk7/cfblk10/cfblk11 ==
  cfblk1 : Inport
  cfblk8 : Inport  Port=2
  cfblk3 : DiscreteFir  SampleTime=1
  cfblk4 : Constant  Value=[-305081804.238437]  SampleTime=1
  cfblk5 : Constant  Value=[-637563579.751119]  SampleTime=1
  cfblk6 : Subsystem
  cfblk7 : Subsystem
  cfblk2 : Outport
  cfblk9 : Outport  Port=2
  wires:
  cfblk1/1 -> cfblk7/1(cfblk1)
  cfblk6/1(cfblk2) -> cfblk3/1
  cfblk3/1 -> cfblk9/1
  cfblk8/1 -> cfblk7/2(cfblk6)
  cfblk6/2(cfblk14) -> cfblk7/3(cfblk7)
  cfblk6/3(cfblk15) -> cfblk7/4(cfblk8)
  cfblk7/1(cfblk2) -> cfblk2/1
  cfblk4/1 -> cfblk6/1(cfblk1)
  cfblk5/1 -> cfblk6/2(cfblk13)

== system Sample594/cfblk7/cfblk10/cfblk12 ==
  cfblk1 : Inport
  cfblk3 : Sum  Inputs=-+
  cfblk4 : Constant  Value=[-822857698.328670]  SampleTime=1
  cfblk5 : Subsystem
  cfblk6 : Subsystem
  cfblk7 : Subsystem
  cfblk8 : Delay  SampleTime=1
  cfblk9 : Delay  SampleTime=1
  cfblk2 : Outport
  wires:
  cfblk7/1(cfblk2) -> cfblk2/1
  cfblk6/1(cfblk2) -> cfblk3/1
  cfblk6/2(cfblk11) -> cfblk5/1(cfblk1)
  cfblk5/1(cfblk2) -> cfblk3/2
  cfblk4/1 -> cfblk5/2(cfblk15)
  cfblk1/1 -> cfblk7/2(cfblk13)
  cfblk7/2(cfblk14) -> cfblk6/2(cfblk9), cfblk6/3(cfblk10)
  cfblk6/3(cfblk12) -> cfblk5/3(cfblk16)
  cfblk3/1 -> cfblk8/1
  cfblk8/1 -> cfblk6/1(cfblk1)
  cfblk5/2(cfblk17) -> cfblk9/1
  cfblk9/1 -> cfblk7/1(cfblk1)

== system Sample594/cfblk7/cfblk10/cfblk13 ==
  cfblk1 : Inport
  cfblk7 : Inport  Port=2
  cfblk8 : Inport  Port=3
  cfblk3 : simulink/Discrete/Transfer Fcn First Order  PoleZ=0.95  ICPrevOutput=0.0  DoSatur=off
  cfblk4 : pid_lib/PID Controller  Controller=PID  Form=Parallel  TimeDomain=Discrete-time  UseExternalTs=off  SampleTime=1  IntegratorMethod=Forward Euler  FilterMethod=Forward Euler  ControllerParametersSource=internal  P=1  I=1  D=0  UseFilter=on  N=100  TunerSelectOption=Transfer Function Based (PID Tuner App)  InitialConditionSource=internal  InitialConditionForIntegrator=0  InitialConditionForFilter=0  DifferentiatorICPrevScaledInput=0  ExternalReset=none  TrackingMode=off  Kt=1  LimitOutput=off  SatLimitsSource=internal  UpperSaturationLimit=inf  LowerSaturationLimit=-inf  LinearizeAsGain=off  AntiWindupMode=none  Kb=1  POutMin=[]  POutMax=[]  IOutMin=[]  IOutMax=[]  DOutMin=[]  DOutMax=[]  NOutMin=[]  NOutMax=[]  SumOutMin=[]  SumOutMax=[]  SaturationOutMin=[]  SaturationOutMax=[]  PParamMin=[]  PParamMax=[]  IParamMin=[]  IParamMax=[]  DParamMin=[]  DParamMax=[]  NParamMin=[]  NParamMax=[]  KbParamMin=[]  KbParamMax=[]  KtParamMin=[]  KtParamMax=[]  KbOutMin=[]  KbOutMax=[]  KtOutMin=[]  KtOutMax=[]  IntegratorOutMin=[]  IntegratorOutMax=[]  FilterOutMin=[]  FilterOutMax=[]  SumI1OutMin=[]  SumI1OutMax=[]  SumI2OutMin=[]  SumI2OutMax=[]  SumI3OutMin=[]  SumI3OutMax=[]  SumI4OutMin=[]  SumI4OutMax=[]  SumDOutMin=[]  SumDOutMax=[]  DifferentiatorOutMin=[]  DifferentiatorOutMax=[]  FilterDiffOutCoefMin=[]  FilterDiffOutCoefMax=[]  ReciprocalOutMin=[]  ReciprocalOutMax=[]  SumDenOutMin=[]  SumDenOutMax=[]  SumNumOutMin=[]  SumNumOutMax=[]  DivideOutMin=[]  DivideOutMax=[]  UdiffTsProdOutMin=[]  UdiffTsProdOutMax=[]  NTsProdOutMin=[]  NTsProdOutMax=[]  UintegralTsProdOutMin=[]  UintegralTsProdOutMax=[]  UngainTsProdOutMin=[]  UngainTsProdOutMax=[]  IntegratorContinuousStateAttributes=''  IntegratorStateMustResolveToSignalObject=off  IntegratorRTWStateStorageClass=Auto  FilterContinuousStateAttributes=''  FilterStateMustResolveToSignalObject=off  FilterRTWStateStorageClass=Auto  ParallelPVariant=InternalParameters  IdealPVariant=Disabled  IVariant=InternalParameters  DVariant=InternalParameters  IntegratorVariant=Discrete  SatVariant=Disabled  AWVariant=Passthrough  PCopyVariant=Disabled  TRVariant=Disabled  FdbkBlocksVariant=Forward  IdealPFdbkVariant=Disabled  SatFdbkVariant=Disabled  DerivativeFilterVariant=ForwardEulerFilter  NVariant=InternalParameters  NCopyVariant=Disabled  FilterICVariant=InternalICsFilter  IntegratorICVariant=InternalICs  ExternalResetVariant=Disabled  TRSumVariant=Passthrough  SumFdbkVariant=Disabled  SumVariant=Sum_PID  TsampFilterVariant=InternalTs  TsampNgainVariant=Passthrough  TsampIntegralVariant=Passthrough  ExternalSaturationOutDataTypeStr=Inherit: Same as second input
  cfblk5 : ComplexToRealImag
  cfblk6 : Subsystem
  cfblk9 : Delay  SampleTime=1
  cfblk2 : Outport
  wires:
  cfblk6/1(cfblk2) -> cfblk3/1
  cfblk1/1 -> cfblk6/1(cfblk1)
  cfblk7/1 -> cfblk2/1
  cfblk3/1 -> cfblk4/1
  cfblk4/1 -> cfblk5/1
  cfblk5/1 -> cfblk9/1
  cfblk9/1 -> cfblk6/2(cfblk12)

== system Sample594/cfblk7/cfblk10/cfblk14 ==
  cfblk1 : Inport
  cfblk{9..13} (5 alike) : Delay  SampleTime=1
  cfblk3 : PermuteDimensions
  cfblk4 : Subsystem
  cfblk5 : Subsystem
  cfblk6 : Subsystem
  cfblk7 : Subsystem
  cfblk2 : Outport
  cfblk8 : Outport  Port=2
  wires:
  cfblk6/1(cfblk2) -> cfblk3/1, cfblk2/1, cfblk13/1
  cfblk1/1 -> cfblk7/1(cfblk1), cfblk4/2(cfblk9), cfblk7/3(cfblk15)
  cfblk7/1(cfblk2) -> cfblk5/2(cfblk12), cfblk6/1(cfblk1), cfblk4/4(cfblk11)
  cfblk5/1(cfblk2) -> cfblk4/1(cfblk1), cfblk8/1, cfblk4/3(cfblk10)
  cfblk4/3(cfblk13) -> cfblk6/2(cfblk11), cfblk11/1
  cfblk4/1(cfblk2) -> cfblk9/1
  cfblk9/1 -> cfblk5/3(cfblk13)
  cfblk4/2(cfblk12) -> cfblk10/1
  cfblk10/1 -> cfblk5/4(cfblk14)
  cfblk11/1 -> cfblk7/2(cfblk14)
  cfblk3/1 -> cfblk12/1
  cfblk12/1 -> cfblk5/1(cfblk1)
  cfblk13/1 -> cfblk5/5(cfblk15)

== system Sample594/cfblk7/cfblk10/cfblk7 ==
  cfblk1 : Inport
  cfblk16 : Inport  Port=2
  cfblk10 : Subsystem
  cfblk11 : Subsystem
  cfblk12 : Subsystem
  cfblk13 : Subsystem
  cfblk14 : Subsystem
  cfblk15 : Subsystem
  cfblk{17..21} (5 alike) : Delay  SampleTime=1
  cfblk3 : Delay  ShowEnablePort=on  SampleTime=1
      settings: InputPortMap=u0,e6
  cfblk4 : Product  Inputs=*
  cfblk5 : simulink/Math Operations/MinMax Running Resettable  Function=min  vinit=0.0
  cfblk6 : Sin  TimeSource=Use external signal  SampleTime=0
  cfblk7 : Reshape
  cfblk8 : Sum  Inputs=+
  cfblk9 : Constant  Value=[874840934.721450]  SampleTime=1
  cfblk2 : Outport
  wires:
  cfblk5/1 -> cfblk4/1, cfblk15/1(cfblk1)
  cfblk13/1(cfblk2) -> cfblk7/1, cfblk15/2(cfblk5)
  cfblk11/1(cfblk2) -> cfblk14/1(cfblk1)
  cfblk12/1(cfblk2) -> cfblk11/1(cfblk1)
  cfblk4/1 -> cfblk10/1(cfblk1), cfblk11/5(cfblk9), cfblk14/4(cfblk7)
  cfblk16/1 -> cfblk8/1, cfblk14/5(cfblk8)
  cfblk9/1 -> cfblk12/1(cfblk1), cfblk14/3(cfblk6)
  cfblk8/1 -> cfblk13/1(cfblk1), cfblk15/3(cfblk6)
  cfblk10/1(cfblk2) -> cfblk3/1
  cfblk3/1 -> cfblk15/4(cfblk7), cfblk15/5(cfblk8), cfblk17/1
  cfblk10/2(cfblk15) -> cfblk11/2(cfblk6)
  cfblk7/1 -> cfblk5/2
  cfblk1/1 -> cfblk13/2(cfblk12), cfblk14/2(cfblk5)
  cfblk15/1(cfblk2) -> cfblk11/3(cfblk7)
  cfblk15/2(cfblk9) -> cfblk6/1
  cfblk10/3(cfblk16) -> cfblk12/2(cfblk8)
  cfblk6/1 -> cfblk2/1, cfblk19/1
  cfblk17/1 -> cfblk10/2(cfblk13)
  cfblk14/1(cfblk2) -> cfblk18/1
  cfblk18/1 -> cfblk11/4(cfblk8)
  cfblk19/1 -> cfblk3/2
  cfblk12/2(cfblk9) -> cfblk20/1
  cfblk20/1 -> cfblk5/1
  cfblk12/3(cfblk10) -> cfblk21/1
  cfblk21/1 -> cfblk10/3(cfblk14)

== system Sample594/cfblk7/cfblk10/cfblk8 ==
  cfblk1 : Inport
  cfblk8 : Inport  Port=2
  cfblk9 : Inport  Port=3
  cfblk10 : Delay  SampleTime=1
  cfblk11 : Delay  SampleTime=1
  cfblk3 : MinMax  Function=max
  cfblk4 : Constant  Value=[-946428797.038929]  SampleTime=1
  cfblk5 : Subsystem
  cfblk6 : Subsystem
  cfblk7 : Subsystem
  cfblk2 : Outport
  wires:
  cfblk1/1 -> cfblk5/1(cfblk1)
  cfblk5/1(cfblk2) -> cfblk6/1(cfblk1)
  cfblk9/1 -> cfblk7/1(cfblk1)
  cfblk6/1(cfblk2) -> cfblk3/1
  cfblk8/1 -> cfblk5/3(cfblk13)
  cfblk4/1 -> cfblk2/1
  cfblk6/2(cfblk8) -> cfblk7/2(cfblk12), cfblk7/4(cfblk14)
  cfblk5/2(cfblk14) -> cfblk7/3(cfblk13)
  cfblk3/1 -> cfblk10/1
  cfblk10/1 -> cfblk6/2(cfblk7)
  cfblk7/1(cfblk2) -> cfblk11/1
  cfblk11/1 -> cfblk5/2(cfblk12)

== system Sample594/cfblk7/cfblk10/cfblk9 ==
  cfblk1 : Inport
  cfblk10 : Inport  Port=2
  cfblk{11..14} (4 alike) : Delay  SampleTime=1
  cfblk3 : simulink/Discrete/Difference  ICPrevInput=0.0  OutMin=[]  OutMax=[]  OutDataTypeStr=Inherit: Inherit via back propagation  OutDataType=fixdt(1, 16)  OutScaling=2^-10  DoSatur=off
  cfblk4 : simulink/Discrete/Difference  ICPrevInput=0.0  OutMin=[]  OutMax=[]  OutDataTypeStr=Inherit: Inherit via back propagation  OutDataType=fixdt(1, 16)  OutScaling=2^-10  DoSatur=off
  cfblk5 : ComplexToMagnitudeAngle
  cfblk6 : Sum  Inputs=-+
  cfblk7 : Subsystem
  cfblk8 : Subsystem
  cfblk9 : Subsystem
  cfblk2 : Outport
  wires:
  cfblk3/1 -> cfblk5/1, cfblk9/4(cfblk13)
  cfblk7/1(cfblk2) -> cfblk4/1
  cfblk4/1 -> cfblk6/2
  cfblk5/2 -> cfblk2/1
  cfblk8/1(cfblk2) -> cfblk7/1(cfblk1), cfblk9/6(cfblk15), cfblk9/7(cfblk16)
  cfblk6/1 -> cfblk3/1, cfblk9/3(cfblk12)
  cfblk1/1 -> cfblk8/2(cfblk6)
  cfblk10/1 -> cfblk9/1(cfblk1), cfblk9/5(cfblk14)
  cfblk7/2(cfblk7) -> cfblk9/2(cfblk11)
  cfblk5/1 -> cfblk11/1
  cfblk11/1 -> cfblk6/1
  cfblk9/1(cfblk2) -> cfblk12/1
  cfblk12/1 -> cfblk8/1(cfblk1)
  cfblk9/2(cfblk17) -> cfblk13/1
  cfblk13/1 -> cfblk8/3(cfblk7)
  cfblk7/3(cfblk8) -> cfblk14/1
  cfblk14/1 -> cfblk8/4(cfblk8)

== system Sample594/cfblk7/cfblk11/cfblk10 ==
  cfblk1 : Inport
  cfblk6 : Inport  Port=2
  cfblk7 : Inport  Port=3
  cfblk3 : simulink/Discrete/Transfer Fcn Real Zero  ZeroZ=0.75  ICPrevInput=0.0  DoSatur=off
      settings: SourceProductBaseCode=SL
  cfblk4 : simulink/Discrete/Difference  ICPrevInput=0.0  OutMin=[]  OutMax=[]  OutDataTypeStr=Inherit: Inherit via back propagation  OutDataType=fixdt(1, 16)  OutScaling=2^-10  DoSatur=off
  cfblk5 : DotProduct  InputSameDT=on  OutDataTypeStr=Inherit: Inherit via internal rule
  cfblk2 : Outport
  wires:
  cfblk1/1 -> cfblk3/1
  cfblk7/1 -> cfblk5/1
  cfblk6/1 -> cfblk5/2
  cfblk3/1 -> cfblk4/1
  cfblk4/1 -> cfblk2/1

== system Sample594/cfblk7/cfblk11/cfblk11 ==
  cfblk1 : Inport
  cfblk9 : Inport  Port=2
  cfblk10 : Delay  SampleTime=1
  cfblk3 : Delay  SampleTime=1
  cfblk4 : MinMax  Function=max  Inputs=2
  cfblk5 : Sum  Inputs=-+
  cfblk6 : Product  Inputs=*
  cfblk7 : Constant  Value=[408238656.679270]  SampleTime=1
  cfblk8 : Subsystem
  cfblk2 : Outport
  wires:
  cfblk4/1 -> cfblk5/1
  cfblk5/1 -> cfblk2/1
  cfblk8/1(cfblk2) -> cfblk3/1
  cfblk6/1 -> cfblk4/1
  cfblk7/1 -> cfblk4/2
  cfblk1/1 -> cfblk8/2(cfblk7)
  cfblk9/1 -> cfblk5/2
  cfblk8/2(cfblk8) -> cfblk6/1
  cfblk3/1 -> cfblk10/1
  cfblk10/1 -> cfblk8/1(cfblk1)

== system Sample594/cfblk7/cfblk11/cfblk9 ==
  cfblk1 : Inport
  cfblk9 : Inport  Port=2
  cfblk10 : Inport  Port=3
  cfblk11 : Inport  Port=4
  cfblk3 : simulink/Discrete/Difference  ICPrevInput=0.0  OutMin=[]  OutMax=[]  OutDataTypeStr=Inherit: Inherit via back propagation  OutDataType=fixdt(1, 16)  OutScaling=2^-10  DoSatur=off
  cfblk4 : Gain  Gain=[58117766.342764]
  cfblk5 : PermuteDimensions
  cfblk6 : Constant  Value=[-630883402.583781]  SampleTime=1
  cfblk7 : Constant  Value=[-559135955.903364]  SampleTime=1
  cfblk8 : Subsystem
  cfblk2 : Outport
  cfblk12 : Outport  Port=2
  wires:
  cfblk11/1 -> cfblk5/1
  cfblk3/1 -> cfblk2/1
  cfblk7/1 -> cfblk4/1
  cfblk6/1 -> cfblk3/1
  cfblk9/1 -> cfblk12/1
  cfblk10/1 -> cfblk8/1(cfblk1)
  cfblk1/1 -> cfblk8/2(cfblk8)
  cfblk4/1 -> cfblk8/3(cfblk9)

== system Sample594/cfblk7/cfblk12/cfblk6 ==
  cfblk1 : Inport
  cfblk14 : Inport  Port=2
  cfblk15 : Inport  Port=3
  cfblk16 : Inport  Port=4
  cfblk10 : Constant  Value=[895973263.071762]  SampleTime=1
  cfblk11 : Subsystem
  cfblk12 : Subsystem
  cfblk13 : Subsystem
  cfblk{17..21} (5 alike) : Delay  SampleTime=1
  cfblk3 : Delay  DelayLengthSource=Input port  SampleTime=1
      settings: InputPortMap=u0,p1
  cfblk4 : DiscreteZeroPole  Poles=[0 0.5]  Gain=1
  cfblk5 : DiscreteIntegrator  ICPrevOutput=DiscIntNeverNeededParam  ICPrevScaledInput=DiscIntNeverNeededParam
  cfblk6 : DiscreteFir  SampleTime=1
  cfblk7 : DiscreteZeroPole  Poles=[0 0.5]  Gain=1
  cfblk8 : Product
  cfblk9 : Sum  Inputs=+-
  cfblk2 : Outport
  wires:
  cfblk12/1(cfblk2) -> cfblk11/1(cfblk1)
  cfblk11/1(cfblk2) -> cfblk2/1
  cfblk12/2(cfblk16) -> cfblk5/1
  cfblk13/1(cfblk2) -> cfblk4/1, cfblk3/2
  cfblk12/3(cfblk17) -> cfblk8/1
  cfblk10/1 -> cfblk12/1(cfblk1)
  cfblk1/1 -> cfblk13/1(cfblk1)
  cfblk5/1 -> cfblk6/1, cfblk21/1
  cfblk7/1 -> cfblk3/1, cfblk17/1
  cfblk14/1 -> cfblk12/2(cfblk11)
  cfblk15/1 -> cfblk9/1
  cfblk8/1 -> cfblk7/1
  cfblk6/1 -> cfblk9/2
  cfblk11/2(cfblk12) -> cfblk8/2, cfblk19/1
  cfblk16/1 -> cfblk12/3(cfblk12)
  cfblk4/1 -> cfblk12/4(cfblk13)
  cfblk17/1 -> cfblk11/3(cfblk11)
  cfblk3/1 -> cfblk18/1
  cfblk18/1 -> cfblk11/2(cfblk10)
  cfblk19/1 -> cfblk12/5(cfblk14)
  cfblk9/1 -> cfblk20/1
  cfblk20/1 -> cfblk13/2(cfblk14)
  cfblk21/1 -> cfblk12/6(cfblk15)

== system Sample594/cfblk7/cfblk12/cfblk7 ==
  cfblk1 : Inport
  cfblk15 : Inport  Port=2
  cfblk16 : Inport  Port=3
  cfblk10 : PermuteDimensions
  cfblk11 : Abs
  cfblk12 : Subsystem
  cfblk13 : Subsystem
  cfblk14 : Subsystem
  cfblk17 : Delay  SampleTime=1
  cfblk18 : Delay  SampleTime=1
  cfblk3 : DiscreteZeroPole  Poles=[0 0.5]  Gain=1
  cfblk4 : DiscreteTransferFcn  SampleTime=1
  cfblk5 : Sqrt  Operator=rSqrt  AlgorithmType=Newton-Raphson  SaturateOnIntegerOverflow=on
  cfblk6 : Sum  Inputs=+
  cfblk7 : Sum
  cfblk8 : Trigonometry
  cfblk9 : Signum
  cfblk2 : Outport
  wires:
  cfblk14/1(cfblk2) -> cfblk10/1
  cfblk5/1 -> cfblk6/1, cfblk13/2(cfblk13), cfblk13/3(cfblk14)
  cfblk13/1(cfblk2) -> cfblk4/1
  cfblk10/1 -> cfblk11/1, cfblk13/4(cfblk15)
  cfblk7/1 -> cfblk12/1(cfblk1)
  cfblk6/1 -> cfblk2/1
  cfblk9/1 -> cfblk5/1
  cfblk11/1 -> cfblk13/1(cfblk1)
  cfblk3/1 -> cfblk8/1
  cfblk15/1 -> cfblk12/3(cfblk10), cfblk14/3(cfblk7)
  cfblk12/1(cfblk2) -> cfblk14/1(cfblk1), cfblk9/1, cfblk14/4(cfblk8)
  cfblk16/1 -> cfblk7/1
  cfblk1/1 -> cfblk3/1
  cfblk8/1 -> cfblk7/2
  cfblk4/1 -> cfblk17/1
  cfblk17/1 -> cfblk14/2(cfblk6)
  cfblk14/2(cfblk9) -> cfblk18/1
  cfblk18/1 -> cfblk12/2(cfblk9)
